simulink model "KiemnghiemDatathudc"  (R2021b)
settings: Solver=VariableStepAuto  StartTime=0.0  StopTime=10  RelTol=1e-3
InitFcn:
  | x_ref = 1; l_ref =0.2; l_ini = 0.6;
  | 
  | %ADRC' s parameter caculation
  | b0 = (ml+mc)/(mc*ml +mc*mt+ml*mt);k_ESO = 70;T_set  = 3;
  | 
  | s_cl = -5.85/T_set;
  | Kp   = s_cl^2;
  | Kd   = -2*s_cl;
  | 
  | s_ESO = k_ESO*s_cl;
  | l1        = -3*s_ESO;
  | l2        = 3*( s_ESO)^2;
  | l3        = -(s_ESO)^3;
  | 
  | %Observer
  | A = [-l1, 1, 0;
  |         -l2, 0, 1;
  |         -l3, 0, 0];
  | B = [0;
  |         b0;
  |         0];
  | L = [l1;
  |        l2;
  |        l3];
  | 
  | b1 = (mt+mc)/(mc*ml +mc*mt+ml*mt);k_ESO1 =100;T_set1  = 3;
  | s_cl1 = -5.85/T_set1;
  | Kp1   = s_cl1^2;
  | Kd1   = -2*s_cl1;
  | 
  | s_ESO1 = k_ESO1*s_cl1;
  | l11        = -3*s_ESO1;
  | l21        = 3*( s_ESO1)^2;
  | l31        = -(s_ESO1)^3;
  | 
  | %Observer
  | A1 = [-l11, 1, 0;
  |         -l21, 0, 1;
  |         -l31, 0, 0];
  | B1 = [0;
  |         b1;
  |         0];
  | L1 = [l11;
  |        l21;
  |        l31];
values from neighbouring files (symbols this model uses):
  g = 9.81    [Thong_so_double_pendulum.m]
undefined symbols (not defined in the file or in its folder): K_pso, mc, sigbuilder_block, T_pso, waof, waol
libraries: neural x95, simulink x11, simulink_extras x11
(part 1 of 6)
settings Model: Creator=Dao Hieu  LastModifiedBy=Admin

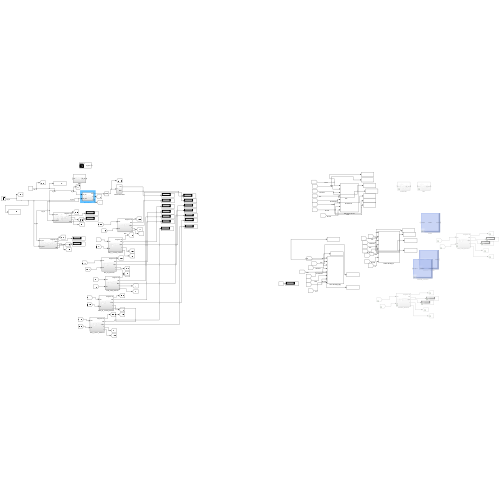
[thumbnail: Simulink's stored preview of the top-level diagram]
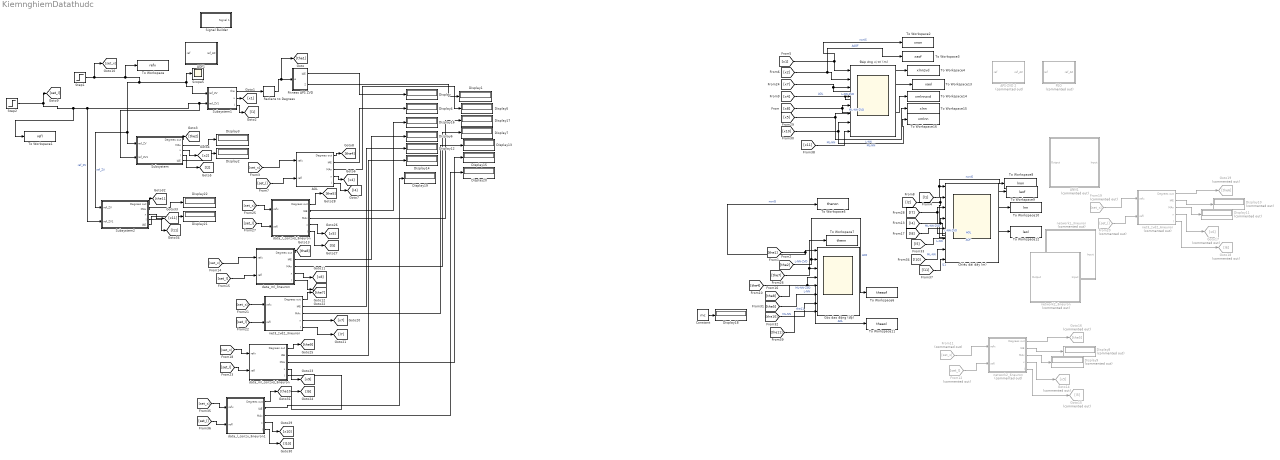
== system KiemnghiemDatathudc ==
  ANN1 : Subsystem  Commented=on
      mask help: Function Fitting Neural Network
      mask Display: e = 0.06;c1 = [120 150 230]/255;c2 = ([120 150 230]+0)/383;c3 = ([120 150 230]+128)/383;patch([0 1 1 0],[0 0 1 1],c1);patch([0 1 1 1-e 1-e 0+e],[0 0 1 1-e 0+e 0+e],c2);patch([0 0 1 1-e 0+e 0+e],[0 1 1 1-e 1-e 0+e],c3);plot([0 1 1 0 0],[0 0 1 1 0]);fprintf('NNET');port_label('input',1,' Input');port_label('output',1,'Output ');
  AOF1 : Subsystem
  AOL : Subsystem
  APS-ZVD 2 : Subsystem  Commented=on
  Chiều dài dây (m) : Scope  NumInputPorts=8
  Constant : Constant  Value=mc
  Display{,1..7,12..22} (19 alike) : Display
  Display{8..11} (4 alike) : Display  Commented=on
  Fitness APS ZVD : Subsystem
  From11 : From  Commented=on  GotoTag=set_x
  From12 : From  Commented=on  GotoTag=set_l
  From19 : From  Commented=on  GotoTag=set_x
  From20 : From  Commented=on  GotoTag=set_l
  Goto14 : Goto  Commented=on  GotoTag=x5
  Goto15 : Goto  Commented=on  GotoTag=l5
  Goto16 : Goto  Commented=on  GotoTag=the5
  Goto17 : Goto  Commented=on  GotoTag=x6
  Goto18 : Goto  Commented=on  GotoTag=l6
  Goto19 : Goto  Commented=on  GotoTag=the6
  Góc dao động (độ) : Scope  NumInputPorts=8
  PSO : Subsystem  Commented=on
  Radians to Degrees : simulink_extras/Transformations/Radians to Degrees
  Scope5 : Scope
  Signal Builder : Subsystem  Tag=STV Subsys  LoadFcn=sigbuilder_block('load');  StartFcn=sigbuilder_block('start');  StopFcn=sigbuilder_block('stop');  ClipboardFcn=sigbuilder_block('clipboard');  mask(Sigbuilder block){tuvar=[0:10]}
      mask help: Simulink:masks:SigbuilderBlock_MD
      mask init:
      | if ~strcmp(get_param(bdroot(gcbh),'SimulationStatus'),'stopped') tuvar = sigbuilder_block('maskInit'); end
      settings: CopyFcn=sigbuilder_block('copy');  DeleteFcn=sigbuilder_block('delete');  ModelCloseFcn=sigbuilder_block('modelClose');  PreSaveFcn=sigbuilder_block('preSave');  PauseFcn=sigbuilder_block('pause');  ContinueFcn=sigbuilder_block('continue');  NameChangeFcn=sigbuilder_block('namechange');  OpenFcn=sigbuilder_block('open',[420.6 144 550.8 400.2 ]);  CloseFcn=sigbuilder_block('close');
      mask Display: plot(0, 0, 100, 100,[2, 2, 32, 32, 2], [68, 8, 8, 68, 68],[32, 2], [38, 38], [32, 19, 2],[53, 60, 44], [32, 17, 17, 2],[16, 16, 31, 31]);txt = getActiveGroup(gcbh);text(2, 100, txt,'verticalAlignment', 'top');
  Step1 : Step  After=x_ref  SampleTime=0
  Step2 : Step  Before=l_ini  After=l_ref  SampleTime=0
  Subsystem : Subsystem
  Subsystem1 : Subsystem
  Subsystem2 : Subsystem
  To Workspace : ToWorkspace  VariableName=refx  SampleTime=0.001
  To Workspace1 : ToWorkspace  VariableName=refl  SampleTime=0.001
  To Workspace10 : ToWorkspace  VariableName=lnn  SampleTime=0.001
  To Workspace11 : ToWorkspace  VariableName=theaol  SampleTime=0.001
  To Workspace12 : ToWorkspace  VariableName=laol  SampleTime=0.001
  To Workspace13 : ToWorkspace  VariableName=xaol  SampleTime=0.001
  To Workspace14 : ToWorkspace  VariableName=xmlnnzvd  SampleTime=0.001
  To Workspace15 : ToWorkspace  VariableName=xlnn  SampleTime=0.001
  To Workspace16 : ToWorkspace  VariableName=xmlnn  SampleTime=0.001
  To Workspace2 : ToWorkspace  VariableName=xnon  SampleTime=0.001
  To Workspace3 : ToWorkspace  VariableName=xaof  SampleTime=0.001
  To Workspace4 : ToWorkspace  VariableName=xlnnzvd  SampleTime=0.001
  To Workspace5 : ToWorkspace  VariableName=thenon  SampleTime=0.001
  To Workspace6 : ToWorkspace  VariableName=theaof  SampleTime=0.001
  To Workspace7 : ToWorkspace  VariableName=thenn  SampleTime=0.001
  To Workspace8 : ToWorkspace  VariableName=lnon  SampleTime=0.001
  To Workspace9 : ToWorkspace  VariableName=laof  SampleTime=0.001
  data_l_conzv_3neuron1 : Subsystem
  data_l_conzvd_3neuron : Subsystem
  data_ml_3neuron : Subsystem
  data_ml_conzvd_3neuron : Subsystem
  net3_zvd2_3neuron : Subsystem
  net3_zvd2_6neuron : Subsystem  Commented=on
  network1_3neuron : Subsystem  Commented=on
      mask help: Custom Neural Network
      mask Display: e = 0.06;c1 = [120 150 230]/255;c2 = ([120 150 230]+0)/383;c3 = ([120 150 230]+128)/383;patch([0 1 1 0],[0 0 1 1],c1);patch([0 1 1 1-e 1-e 0+e],[0 0 1 1-e 0+e 0+e],c2);patch([0 0 1 1-e 0+e 0+e],[0 1 1 1-e 1-e 0+e],c3);plot([0 1 1 0 0],[0 0 1 1 0]);fprintf('NNET');port_label('input',1,' Input');port_label('output',1,'Output ');
  network2_3neuron : Subsystem  Commented=on
      mask help: Custom Neural Network
      mask Display: e = 0.06;c1 = [120 150 230]/255;c2 = ([120 150 230]+0)/383;c3 = ([120 150 230]+128)/383;patch([0 1 1 0],[0 0 1 1],c1);patch([0 1 1 1-e 1-e 0+e],[0 0 1 1-e 0+e 0+e],c2);patch([0 0 1 1-e 0+e 0+e],[0 1 1 1-e 1-e 0+e],c3);plot([0 1 1 0 0],[0 0 1 1 0]);fprintf('NNET');port_label('input',1,' Input');port_label('output',1,'Output ');
  network2_6neuron : Subsystem  Commented=on
  Đáp ứng vị trí (m) : Scope  NumInputPorts=8
  wires:
  Radians to Degrees/1 -> [the1], Fitness APS ZVD/1(e)
  Fitness APS ZVD/2(MAx) -> Display1/1
  Fitness APS ZVD/1(IAE) -> Display/1
  Subsystem1/1(the) -> Radians to Degrees/1
  [x2] -> Đáp ứng vị trí (m)/2, To Workspace3/1  "AAOF"
  [x1] -> To Workspace2/1, Đáp ứng vị trí (m)/1  "nonIS"
  [the2] -> To Workspace6/1, Góc dao động (độ)/2  "AOF"
  [the1] -> To Workspace5/1, Góc dao động (độ)/1  "nonIS"
  [l2] -> To Workspace9/1, Chiều dài dây (m)/2  "AOF"
  [l1] -> To Workspace8/1, Chiều dài dây (m)/1  "nonIS"
  Subsystem1/2(x) -> [x1]
  Subsystem1/3(l) -> [l1]
  From11/1 -> network2_6neuron/1(refx)
  network2_6neuron/1(Degrees out) -> Goto16/1
  network2_6neuron/2(IAE) -> Display8/1
  network2_6neuron/3(MAx) -> Display9/1
  network2_6neuron/4(x) -> Goto14/1
  network2_6neuron/5(l) -> Goto15/1
  From12/1 -> network2_6neuron/2(refl)
  net3_zvd2_6neuron/5(l) -> Goto18/1
  net3_zvd2_6neuron/1(Degrees out) -> Goto19/1
  net3_zvd2_6neuron/4(x) -> Goto17/1
  net3_zvd2_6neuron/3(MAx) -> Display11/1
  net3_zvd2_6neuron/2(IAE) -> Display10/1
  From19/1 -> net3_zvd2_6neuron/1(refx)
  From20/1 -> net3_zvd2_6neuron/2(refl)
  net3_zvd2_3neuron/5(l) -> [l7]
  net3_zvd2_3neuron/1(Degrees out) -> [the7]
  net3_zvd2_3neuron/4(x) -> [x7]
  net3_zvd2_3neuron/3(MAx) -> Display13/1
  net3_zvd2_3neuron/2(IAE) -> Display12/1
  [set_x] -> net3_zvd2_3neuron/1(refx)
  [set_l] -> net3_zvd2_3neuron/2(refl)
  [x7] -> To Workspace4/1, Đáp ứng vị trí (m)/3  "L-NN-ZVD"
  [l7] -> To Workspace10/1, Chiều dài dây (m)/3  "L-NN-ZVD"
  [the7] -> To Workspace7/1, Góc dao động (độ)/3  "L-NN-ZVD"
  AOL/2(IAE) -> Display4/1
  AOL/4(x) -> [x4]
  AOL/5(l) -> [l4]
  AOL/3(MAx) -> Display5/1
  [set_l] -> AOL/2(refl)
  AOL/1(Degrees out) -> [the4]
  [set_x] -> AOL/1(refx)
  [x4] -> To Workspace13/1, Đáp ứng vị trí (m)/4  "AOL"
  [the4] -> To Workspace11/1, Góc dao động (độ)/4  "AOL"
  [l4] -> To Workspace12/1, Chiều dài dây (m)/4  "AOL"
  [set_l] -> data_ml_3neuron/2(refl)
  [set_x] -> data_ml_3neuron/1(refx)
  data_ml_3neuron/1(Degrees out) -> [the8]
  data_ml_3neuron/3(MAx) -> Display7/1
  data_ml_3neuron/5(l) -> [l8]
  data_ml_3neuron/2(IAE) -> Display6/1
  data_ml_3neuron/4(x) -> [x8]
  [x8] -> To Workspace14/1, Đáp ứng vị trí (m)/5  "ML-NN-ZVD"
  [the8] -> Góc dao động (độ)/5  "ML-NN-ZVD"
  [l8] -> Chiều dài dây (m)/5  "ML-NN-ZVD"
  [set_l] -> data_ml_conzvd_3neuron/2(refl)
  [set_x] -> data_ml_conzvd_3neuron/1(refx)
  data_ml_conzvd_3neuron/1(Degrees out) -> [the9]
  data_ml_conzvd_3neuron/3(MAx) -> Display15/1
  data_ml_conzvd_3neuron/5(l) -> [l9]
  data_ml_conzvd_3neuron/2(IAE) -> Display14/1
  data_ml_conzvd_3neuron/4(x) -> [x9]
  [set_l] -> data_l_conzvd_3neuron/2(refl)
  [set_x] -> data_l_conzvd_3neuron/1(refx)
  data_l_conzvd_3neuron/1(Degrees out) -> [the5]
  data_l_conzvd_3neuron/3(MAx) -> Display17/1
  data_l_conzvd_3neuron/5(l) -> [l5]
  data_l_conzvd_3neuron/2(IAE) -> Display16/1
  data_l_conzvd_3neuron/4(x) -> [x5]
  [l5] -> Chiều dài dây (m)/6  "L-NN"
  [l10] -> Chiều dài dây (m)/7  "ML-NN"
  [the5] -> Góc dao động (độ)/6  "L-NN"
  [the10] -> Góc dao động (độ)/7  "ML-NN"
  [x5] -> To Workspace15/1, Đáp ứng vị trí (m)/6  "L-NN"
  [x10] -> To Workspace16/1, Đáp ứng vị trí (m)/7  "ML-NN"
  Constant/1 -> Display18/1
  data_l_conzv_3neuron1/5(l) -> [l10]
  data_l_conzv_3neuron1/2(IAE) -> Display19/1
  data_l_conzv_3neuron1/4(x) -> [x10]
  [set_x] -> data_l_conzv_3neuron1/1(refx)
  [set_l] -> data_l_conzv_3neuron1/2(refl)
  data_l_conzv_3neuron1/1(Degrees out) -> [the10]
  data_l_conzv_3neuron1/3(MAx) -> Display20/1
  Subsystem/1(Degrees out) -> [the2]
  Subsystem/2(MAx) -> Display3/1
  Subsystem/3(x) -> [x2]
  Subsystem/4(l) -> [l2]
  Subsystem/5(IAE) -> Display2/1
  Subsystem2/4(l) -> [l11]
  Subsystem2/1(Degrees out) -> [the11]
  Step1/1 -> To Workspace/1, Subsystem2/1(ref_ZV), Subsystem/1(ref_ZV), Subsystem1/1(ref_ZV), Scope5/1, [set_x]  "ref_ZV"
  Step2/1 -> Subsystem/2(ref_ZV1), Subsystem1/2(ref_ZV1), Subsystem2/2(ref_ZV1), To Workspace1/1, [set_l]  "ref_ZV"
  Subsystem2/2(MAx) -> Display22/1
  Subsystem2/3(x) -> [x11]
  Subsystem2/5(IAE) -> Display21/1
  [l11] -> Chiều dài dây (m)/8  "l11"
  [x11] -> Đáp ứng vị trí (m)/8  "ML-NN"
  [the11] -> Góc dao động (độ)/8  "the11"

== system KiemnghiemDatathudc/ANN1 ==
  Input : Inport  PortDimensions=1
      mask Display: e = 0.06;c1 = [120 230 180]/255;c2 = ([120 230 180]+0)/(256+128);c3 = ([120 230 180]+128)/(256+128);patch([0 1 1 0],[0 0 1 1],c1);patch([0 1 1 1-e 1-e 0+e],[0 0 1 1-e 0+e 0+e],c2);patch([0 0 1 1-e 0+e 0+e],[0 1 1 1-e 1-e 0+e],c3);plot([0 1 1 0 0],[0 0 1 1 0]);
  Layer 1 : Subsystem
      mask Display: e = 0.06;c1 = [120 150 230]/255;c2 = ([120 150 230]+0)/383;c3 = ([120 150 230]+128)/383;patch([0 1 1 0],[0 0 1 1],c1);patch([0 1 1 1-e 1-e 0+e],[0 0 1 1-e 0+e 0+e],c2);patch([0 0 1 1-e 0+e 0+e],[0 1 1 1-e 1-e 0+e],c3);plot([0 1 1 0 0],[0 0 1 1 0]);
  Layer 2 : Subsystem
      mask Display: e = 0.06;c1 = [120 150 230]/255;c2 = ([120 150 230]+0)/383;c3 = ([120 150 230]+128)/383;patch([0 1 1 0],[0 0 1 1],c1);patch([0 1 1 1-e 1-e 0+e],[0 0 1 1-e 0+e 0+e],c2);patch([0 0 1 1-e 0+e 0+e],[0 1 1 1-e 1-e 0+e],c3);plot([0 1 1 0 0],[0 0 1 1 0]);
  Process Input 1 : Subsystem
      mask Display: e = 0.06;c1 = [120 150 230]/255;c2 = ([120 150 230]+0)/383;c3 = ([120 150 230]+128)/383;patch([0 1 1 0],[0 0 1 1],c1);patch([0 1 1 1-e 1-e 0+e],[0 0 1 1-e 0+e 0+e],c2);patch([0 0 1 1-e 0+e 0+e],[0 1 1 1-e 1-e 0+e],c3);plot([0 1 1 0 0],[0 0 1 1 0]);
  Process Output 1 : Subsystem
      mask Display: e = 0.06;c1 = [120 150 230]/255;c2 = ([120 150 230]+0)/383;c3 = ([120 150 230]+128)/383;patch([0 1 1 0],[0 0 1 1],c1);patch([0 1 1 1-e 1-e 0+e],[0 0 1 1-e 0+e 0+e],c2);patch([0 0 1 1-e 0+e 0+e],[0 1 1 1-e 1-e 0+e],c3);plot([0 1 1 0 0],[0 0 1 1 0]);
  Output : Outport  InitialOutput=[0;0]
      mask Display: e = 0.06;c1 = [120 230 180]/255;c2 = ([120 230 180]+0)/(256+128);c3 = ([120 230 180]+128)/(256+128);patch([0 1 1 0],[0 0 1 1],c1);patch([0 1 1 1-e 1-e 0+e],[0 0 1 1-e 0+e 0+e],c2);patch([0 0 1 1-e 0+e 0+e],[0 1 1 1-e 1-e 0+e],c3);plot([0 1 1 0 0],[0 0 1 1 0]);
  wires:
  Input/1 -> Process Input 1/1(x)
  Process Output 1/1(y) -> Output/1
  Process Input 1/1(p) -> Layer 1/1("p{1}")
  Layer 1/1("a{1}") -> [feedback1]
  [feedback1] -> Layer 2/1("a{1} ")
  Layer 2/1("a{2}") -> Process Output 1/1(a)

== system KiemnghiemDatathudc/AOF1 ==
  ref : Inport
  Gain : Gain  Gain=0.5
  Gain1 : Gain  Gain=0.5
  Sum : Sum
  Transport Delay : TransportDelay  DelayTime=pi/sqrt(g/0.4)
  ref_AZ : Outport
  wires:
  Gain1/1 -> Transport Delay/1
  Gain/1 -> Sum/1
  Transport Delay/1 -> Sum/2
  Sum/1 -> ref_AZ/1
  ref/1 -> Gain/1, Gain1/1

== system KiemnghiemDatathudc/AOL ==
  refx : Inport
  refl : Inport  Port=2
  AOL : Subsystem
  Fitness APS ZVD4 : Subsystem
  Radians to Degrees4 : simulink_extras/Transformations/Radians to Degrees
  Subsystem5 : Subsystem
  Degrees out : Outport
  IAE : Outport  Port=2
  MAx : Outport  Port=3
  x : Outport  Port=4
  l : Outport  Port=5
  wires:
  refl/1 -> Subsystem5/2(ref_ZV1)
  Subsystem5/1(the) -> Radians to Degrees4/1
  Fitness APS ZVD4/1(IAE) -> IAE/1
  Radians to Degrees4/1 -> Degrees out/1, Fitness APS ZVD4/1(e)
  Subsystem5/3(l) -> l/1
  AOL/1(ref_AZ) -> Subsystem5/1(ref_ZV)  "ref_ZV"
  refx/1 -> AOL/1(ref)
  Subsystem5/2(x) -> x/1
  Fitness APS ZVD4/2(MAx) -> MAx/1

== system KiemnghiemDatathudc/APS-ZVD 2 ==
  ref : Inport
  Gain : Gain
  Gain1 : Gain  Gain=-1
  Gain2 : Gain
  Sum : Sum  Inputs=+++
  Transport Delay : TransportDelay  DelayTime=0.213149037770351
  Transport Delay1 : TransportDelay  DelayTime=0.426777072460345
  ref_AZ : Outport
  wires:
  Gain1/1 -> Transport Delay/1
  Gain/1 -> Sum/1
  Transport Delay/1 -> Sum/2
  Sum/1 -> ref_AZ/1
  ref/1 -> Gain/1, Gain2/1, Gain1/1
  Gain2/1 -> Transport Delay1/1
  Transport Delay1/1 -> Sum/3

== system KiemnghiemDatathudc/Fitness APS ZVD ==
  e : Inport
  Abs : Abs
  Abs1 : Abs
  Integrator : Integrator
  MinMax Running Resettable : simulink/Math Operations/MinMax Running Resettable  Function=max  vinit=0.0
  Step : Step  Time=0.000001  Before=1  After=0  SampleTime=0
  IAE : Outport
  MAx : Outport  Port=2
  wires:
  Abs/1 -> Integrator/1
  Abs1/1 -> MinMax Running Resettable/1
  Step/1 -> MinMax Running Resettable/2
  e/1 -> Abs/1, Abs1/1
  Integrator/1 -> IAE/1
  MinMax Running Resettable/1 -> MAx/1

== system KiemnghiemDatathudc/PSO ==
  ref : Inport
  Gain : Gain  Gain=1/(K_pso^2+2*K_pso+1)
  Gain1 : Gain  Gain=2*K_pso/(K_pso^2+2*K_pso+1)
  Gain2 : Gain  Gain=K_pso^2/(K_pso^2+2*K_pso+1)
  Sum : Sum  Inputs=+++
  Transport Delay : TransportDelay  DelayTime=T_pso
  Transport Delay1 : TransportDelay  DelayTime=2*T_pso
  ref_AZ : Outport
  wires:
  Gain1/1 -> Transport Delay/1
  Gain/1 -> Sum/1
  Transport Delay/1 -> Sum/2
  Sum/1 -> ref_AZ/1
  ref/1 -> Gain/1, Gain2/1, Gain1/1
  Gain2/1 -> Transport Delay1/1
  Transport Delay1/1 -> Sum/3

== system KiemnghiemDatathudc/Signal Builder ==
  Demux : Demux  Tag=STV Demux  Outputs=1
      settings: DisplayOption=none
  FromWs : FromWorkspace  Tag=STV FromWs  VariableName=tuvar
      SigBuilderData=|
      | common.afterFinalStr = 'Extrapolate'
      | common.sampleTime = 0
      | dataSet.timeRange = [0 10]
      | dataSet.name = 'Group 1'
      | sbobj.Groups.Name = 'Group 1'
      | sbobj.Groups.Signals.Name = 'Signal 1'
      | sbobj.Groups.Signals.XData = [0 1 1 3 3 10]
      | sbobj.Groups.Signals.YData = [0.6 0.6 0.2 0.2 0.6 0.6]
  Signal 1 : Outport  Tag=STV Outport
  wires:
  Demux/1 -> Signal 1/1
  FromWs/1 -> Demux/1

== system KiemnghiemDatathudc/Subsystem ==
  ref_ZV : Inport
  ref_ZV1 : Inport  Port=2
  AOF : Subsystem
  AOF2 : Subsystem
  Constant : Constant  Value=l_ini
  Constant1 : Constant  Value=l_ini
  Fitness APS ZVD1 : Subsystem
  Radians to Degrees1 : simulink_extras/Transformations/Radians to Degrees
  Scope : Scope  NumInputPorts=2
  Subsystem5 : Subsystem
  Subtract : Sum  Inputs=+-
  Sum : Sum  Inputs=|++
  Degrees out : Outport
  MAx : Outport  Port=2
  x : Outport  Port=3
  l : Outport  Port=4
  IAE : Outport  Port=5
  wires:
  Radians to Degrees1/1 -> Degrees out/1, Fitness APS ZVD1/1(e)
  Subsystem5/2(x) -> x/1
  ref_ZV1/1 -> Subtract/1, Scope/1
  Subsystem5/3(l) -> l/1
  Subsystem5/1(the) -> Radians to Degrees1/1
  AOF2/1(ref_AZ) -> Sum/1  "ref_ZV"
  AOF/1(ref_AZ) -> Subsystem5/1(ref_ZV)  "ref_ZV"
  Fitness APS ZVD1/1(IAE) -> IAE/1
  Fitness APS ZVD1/2(MAx) -> MAx/1
  ref_ZV/1 -> AOF/1(ref)
  Subtract/1 -> AOF2/1(ref)
  Constant/1 -> Subtract/2
  Sum/1 -> Subsystem5/2(ref_ZV1), Scope/2
  Constant1/1 -> Sum/2

== system KiemnghiemDatathudc/Subsystem1 ==
  ref_ZV : Inport
  ref_ZV1 : Inport  Port=2
  "ADRC " : Subsystem
  ADRC 1 : Subsystem
  Constant : Constant  Value=mc
  Gain : Gain  Gain=1/3
  Subsystem : Subsystem
  the : Outport
  x : Outport  Port=2
  l : Outport  Port=3
  wires:
  Subsystem/1(x) -> x/1, "ADRC "/2(x)  "Position"
  ADRC 1/1(u) -> Subsystem/2(ul)  "ADRC"
  Subsystem/3(the) -> Gain/1
  Subsystem/2(l) -> ADRC 1/2(x), l/1  "Length"
  "ADRC "/1(u) -> Subsystem/1(ut)  "ADRC"
  ref_ZV1/1 -> ADRC 1/1(ref)
  ref_ZV/1 -> "ADRC "/1(ref)
  Gain/1 -> the/1
  Constant/1 -> Subsystem/3(mc)

== system KiemnghiemDatathudc/Subsystem2 ==
  ref_ZV : Inport
  ref_ZV1 : Inport  Port=2
  AOF : Subsystem
  Fitness APS ZVD1 : Subsystem
  Radians to Degrees1 : simulink_extras/Transformations/Radians to Degrees
  Subsystem5 : Subsystem
  Degrees out : Outport
  MAx : Outport  Port=2
  x : Outport  Port=3
  l : Outport  Port=4
  IAE : Outport  Port=5
  wires:
  Radians to Degrees1/1 -> Degrees out/1, Fitness APS ZVD1/1(e)
  Subsystem5/2(x) -> x/1
  Subsystem5/3(l) -> l/1
  Subsystem5/1(the) -> Radians to Degrees1/1
  ref_ZV1/1 -> Subsystem5/2(ref_ZV1)  "ref_ZV"
  AOF/1(ref_AZ) -> Subsystem5/1(ref_ZV)  "ref_ZV"
  Fitness APS ZVD1/1(IAE) -> IAE/1
  Fitness APS ZVD1/2(MAx) -> MAx/1
  ref_ZV/1 -> AOF/1(ref)

== system KiemnghiemDatathudc/data_l_conzv_3neuron1 ==
  refx : Inport
  refl : Inport  Port=2
  Custom Neural Network1 : Subsystem
      mask help: Custom Neural Network
      mask Display: e = 0.06;c1 = [120 150 230]/255;c2 = ([120 150 230]+0)/383;c3 = ([120 150 230]+128)/383;patch([0 1 1 0],[0 0 1 1],c1);patch([0 1 1 1-e 1-e 0+e],[0 0 1 1-e 0+e 0+e],c2);patch([0 0 1 1-e 0+e 0+e],[0 1 1 1-e 1-e 0+e],c3);plot([0 1 1 0 0],[0 0 1 1 0]);fprintf('NNET');port_label('input',1,' Input');port_label('output',1,'Output ');
  Fitness APS ZVD4 : Subsystem
  Radians to Degrees4 : simulink_extras/Transformations/Radians to Degrees
  Scope : Scope
  Subsystem5 : Subsystem
  ZV3 : Subsystem
  Degrees out : Outport
  IAE : Outport  Port=2
  MAx : Outport  Port=3
  x : Outport  Port=4
  l : Outport  Port=5
  wires:
  refl/1 -> Subsystem5/2(ref_ZV1)
  Subsystem5/1(the) -> Radians to Degrees4/1
  Fitness APS ZVD4/1(IAE) -> IAE/1
  Radians to Degrees4/1 -> Degrees out/1, Fitness APS ZVD4/1(e)
  Subsystem5/3(l) -> Custom Neural Network1/1(Input), l/1
  ZV3/1(ref_AZ) -> Scope/1, Subsystem5/1(ref_ZV)  "ref_ZV"
  refx/1 -> ZV3/1(ref)
  Subsystem5/2(x) -> x/1
  Fitness APS ZVD4/2(MAx) -> MAx/1
  Custom Neural Network1/1(Output) -> ZV3/2(Input)

== system KiemnghiemDatathudc/data_l_conzvd_3neuron ==
  refx : Inport
  refl : Inport  Port=2
  Custom Neural Network : Subsystem
      mask help: Custom Neural Network
      mask Display: e = 0.06;c1 = [120 150 230]/255;c2 = ([120 150 230]+0)/383;c3 = ([120 150 230]+128)/383;patch([0 1 1 0],[0 0 1 1],c1);patch([0 1 1 1-e 1-e 0+e],[0 0 1 1-e 0+e 0+e],c2);patch([0 0 1 1-e 0+e 0+e],[0 1 1 1-e 1-e 0+e],c3);plot([0 1 1 0 0],[0 0 1 1 0]);fprintf('NNET');port_label('input',1,' Input');port_label('output',1,'Output ');
  Demux2 : Demux  Outputs=2
  Fitness APS ZVD4 : Subsystem
  Radians to Degrees4 : simulink_extras/Transformations/Radians to Degrees
  Subsystem5 : Subsystem
  ZVD3 : Subsystem
  Degrees out : Outport
  IAE : Outport  Port=2
  MAx : Outport  Port=3
  x : Outport  Port=4
  l : Outport  Port=5
  wires:
  refl/1 -> Subsystem5/2(ref_ZV1)
  Subsystem5/1(the) -> Radians to Degrees4/1
  Fitness APS ZVD4/1(IAE) -> IAE/1
  Radians to Degrees4/1 -> Degrees out/1, Fitness APS ZVD4/1(e)
  Subsystem5/3(l) -> ZVD3/4(Input1), Custom Neural Network/1(Input), l/1
  Demux2/1 -> ZVD3/2(Input)
  ZVD3/1(ref_AZ) -> Subsystem5/1(ref_ZV)  "ref_ZV"
  Demux2/2 -> ZVD3/3(Input2)
  Custom Neural Network/1(Output) -> Demux2/1
  refx/1 -> ZVD3/1(ref)
  Subsystem5/2(x) -> x/1
  Fitness APS ZVD4/2(MAx) -> MAx/1

== system KiemnghiemDatathudc/data_ml_3neuron ==
  refx : Inport
  refl : Inport  Port=2
  Constant : Constant  Value=mc
  Custom Neural Network : Subsystem
      mask help: Custom Neural Network
      mask Display: e = 0.06;c1 = [120 150 230]/255;c2 = ([120 150 230]+0)/383;c3 = ([120 150 230]+128)/383;patch([0 1 1 0],[0 0 1 1],c1);patch([0 1 1 1-e 1-e 0+e],[0 0 1 1-e 0+e 0+e],c2);patch([0 0 1 1-e 0+e 0+e],[0 1 1 1-e 1-e 0+e],c3);plot([0 1 1 0 0],[0 0 1 1 0]);fprintf('NNET');port_label('input',1,' Input');port_label('output',1,'Output ');
  Demux2 : Demux  Outputs=2
  Fitness APS ZVD4 : Subsystem
  Mux : Mux  Inputs=2
  Radians to Degrees4 : simulink_extras/Transformations/Radians to Degrees
  Subsystem5 : Subsystem
  ZVD3 : Subsystem
  Degrees out : Outport
  IAE : Outport  Port=2
  MAx : Outport  Port=3
  x : Outport  Port=4
  l : Outport  Port=5
  wires:
  refl/1 -> Subsystem5/2(ref_ZV1)
  Subsystem5/1(the) -> Radians to Degrees4/1
  Fitness APS ZVD4/1(IAE) -> IAE/1
  Radians to Degrees4/1 -> Degrees out/1, Fitness APS ZVD4/1(e)
  Subsystem5/3(l) -> Mux/2, l/1
  Demux2/1 -> ZVD3/2(K)
  ZVD3/1(ref_AZ) -> Subsystem5/1(ref_ZV)  "ref_ZV"
  Demux2/2 -> ZVD3/3(T)
  Custom Neural Network/1(Output) -> Demux2/1
  refx/1 -> ZVD3/1(ref)
  Subsystem5/2(x) -> x/1
  Fitness APS ZVD4/2(MAx) -> MAx/1
  Mux/1 -> Custom Neural Network/1(Input)
  Constant/1 -> Mux/1

== system KiemnghiemDatathudc/data_ml_conzvd_3neuron ==
  refx : Inport
  refl : Inport  Port=2
  Constant : Constant  Value=mc
  Custom Neural Network : Subsystem
      mask help: Custom Neural Network
      mask Display: e = 0.06;c1 = [120 150 230]/255;c2 = ([120 150 230]+0)/383;c3 = ([120 150 230]+128)/383;patch([0 1 1 0],[0 0 1 1],c1);patch([0 1 1 1-e 1-e 0+e],[0 0 1 1-e 0+e 0+e],c2);patch([0 0 1 1-e 0+e 0+e],[0 1 1 1-e 1-e 0+e],c3);plot([0 1 1 0 0],[0 0 1 1 0]);fprintf('NNET');port_label('input',1,' Input');port_label('output',1,'Output ');
  Demux2 : Demux  Outputs=2
  Fitness APS ZVD4 : Subsystem
  Mux : Mux  Inputs=2
  Radians to Degrees4 : simulink_extras/Transformations/Radians to Degrees
  Subsystem5 : Subsystem
  ZVD3 : Subsystem
  Degrees out : Outport
  IAE : Outport  Port=2
  MAx : Outport  Port=3
  x : Outport  Port=4
  l : Outport  Port=5
  wires:
  refl/1 -> Subsystem5/2(ref_ZV1)
  Subsystem5/1(the) -> Radians to Degrees4/1
  Fitness APS ZVD4/1(IAE) -> IAE/1
  Radians to Degrees4/1 -> Degrees out/1, Fitness APS ZVD4/1(e)
  Subsystem5/3(l) -> Mux/2, l/1
  Demux2/1 -> ZVD3/2(Input)
  ZVD3/1(ref_AZ) -> Subsystem5/1(ref_ZV)  "ref_ZV"
  Demux2/2 -> ZVD3/3(Input1)
  Custom Neural Network/1(Output) -> Demux2/1
  refx/1 -> ZVD3/1(ref)
  Subsystem5/2(x) -> x/1
  Fitness APS ZVD4/2(MAx) -> MAx/1
  Mux/1 -> Custom Neural Network/1(Input)
  Constant/1 -> Mux/1

== system KiemnghiemDatathudc/net3_zvd2_3neuron ==
  refx : Inport
  refl : Inport  Port=2
  Demux2 : Demux  Outputs=2
  Fitness APS ZVD4 : Subsystem
  Radians to Degrees4 : simulink_extras/Transformations/Radians to Degrees
  Scope : Scope
  Subsystem5 : Subsystem
  ZVD3 : Subsystem
  net3_zvd2_3neuron : Subsystem
      mask help: Custom Neural Network
      mask Display: e = 0.06;c1 = [120 150 230]/255;c2 = ([120 150 230]+0)/383;c3 = ([120 150 230]+128)/383;patch([0 1 1 0],[0 0 1 1],c1);patch([0 1 1 1-e 1-e 0+e],[0 0 1 1-e 0+e 0+e],c2);patch([0 0 1 1-e 0+e 0+e],[0 1 1 1-e 1-e 0+e],c3);plot([0 1 1 0 0],[0 0 1 1 0]);fprintf('NNET');port_label('input',1,' Input');port_label('output',1,'Output ');
  Degrees out : Outport
  IAE : Outport  Port=2
  MAx : Outport  Port=3
  x : Outport  Port=4
  l : Outport  Port=5
  wires:
  refl/1 -> Subsystem5/2(ref_ZV1)
  Subsystem5/1(the) -> Radians to Degrees4/1
  Fitness APS ZVD4/1(IAE) -> IAE/1
  Radians to Degrees4/1 -> Degrees out/1, Fitness APS ZVD4/1(e)
  Subsystem5/3(l) -> net3_zvd2_3neuron/1(Input), l/1
  Demux2/1 -> ZVD3/2(K)
  ZVD3/1(ref_AZ) -> Scope/1, Subsystem5/1(ref_ZV)  "ref_ZV"
  Demux2/2 -> ZVD3/3(T)
  net3_zvd2_3neuron/1(Output) -> Demux2/1
  refx/1 -> ZVD3/1(ref)
  Subsystem5/2(x) -> x/1
  Fitness APS ZVD4/2(MAx) -> MAx/1

== system KiemnghiemDatathudc/net3_zvd2_6neuron ==
  refx : Inport
  refl : Inport  Port=2
  Demux2 : Demux  Outputs=2
  Fitness APS ZVD4 : Subsystem
  Radians to Degrees4 : simulink_extras/Transformations/Radians to Degrees
  Subsystem5 : Subsystem
  ZVD3 : Subsystem
  net3_zvd2_6neuron : Subsystem
      mask help: Custom Neural Network
      mask Display: e = 0.06;c1 = [120 150 230]/255;c2 = ([120 150 230]+0)/383;c3 = ([120 150 230]+128)/383;patch([0 1 1 0],[0 0 1 1],c1);patch([0 1 1 1-e 1-e 0+e],[0 0 1 1-e 0+e 0+e],c2);patch([0 0 1 1-e 0+e 0+e],[0 1 1 1-e 1-e 0+e],c3);plot([0 1 1 0 0],[0 0 1 1 0]);fprintf('NNET');port_label('input',1,' Input');port_label('output',1,'Output ');
  Degrees out : Outport
  IAE : Outport  Port=2
  MAx : Outport  Port=3
  x : Outport  Port=4
  l : Outport  Port=5
  wires:
  refl/1 -> Subsystem5/2(ref_ZV1)
  Subsystem5/1(the) -> Radians to Degrees4/1
  Fitness APS ZVD4/1(IAE) -> IAE/1
  Radians to Degrees4/1 -> Degrees out/1, Fitness APS ZVD4/1(e)
  Subsystem5/3(l) -> net3_zvd2_6neuron/1(Input), l/1
  Demux2/1 -> ZVD3/2(K)
  ZVD3/1(ref_AZ) -> Subsystem5/1(ref_ZV)  "ref_ZV"
  Demux2/2 -> ZVD3/3(T)
  net3_zvd2_6neuron/1(Output) -> Demux2/1
  refx/1 -> ZVD3/1(ref)
  Subsystem5/2(x) -> x/1
  Fitness APS ZVD4/2(MAx) -> MAx/1

== system KiemnghiemDatathudc/network1_3neuron ==
  Input : Inport  PortDimensions=1
      mask Display: e = 0.06;c1 = [120 230 180]/255;c2 = ([120 230 180]+0)/(256+128);c3 = ([120 230 180]+128)/(256+128);patch([0 1 1 0],[0 0 1 1],c1);patch([0 1 1 1-e 1-e 0+e],[0 0 1 1-e 0+e 0+e],c2);patch([0 0 1 1-e 0+e 0+e],[0 1 1 1-e 1-e 0+e],c3);plot([0 1 1 0 0],[0 0 1 1 0]);
  Layer 1 : Subsystem
      mask Display: e = 0.06;c1 = [120 150 230]/255;c2 = ([120 150 230]+0)/383;c3 = ([120 150 230]+128)/383;patch([0 1 1 0],[0 0 1 1],c1);patch([0 1 1 1-e 1-e 0+e],[0 0 1 1-e 0+e 0+e],c2);patch([0 0 1 1-e 0+e 0+e],[0 1 1 1-e 1-e 0+e],c3);plot([0 1 1 0 0],[0 0 1 1 0]);
  Layer 2 : Subsystem
      mask Display: e = 0.06;c1 = [120 150 230]/255;c2 = ([120 150 230]+0)/383;c3 = ([120 150 230]+128)/383;patch([0 1 1 0],[0 0 1 1],c1);patch([0 1 1 1-e 1-e 0+e],[0 0 1 1-e 0+e 0+e],c2);patch([0 0 1 1-e 0+e 0+e],[0 1 1 1-e 1-e 0+e],c3);plot([0 1 1 0 0],[0 0 1 1 0]);
  Process Input 1 : Subsystem
      mask Display: e = 0.06;c1 = [120 150 230]/255;c2 = ([120 150 230]+0)/383;c3 = ([120 150 230]+128)/383;patch([0 1 1 0],[0 0 1 1],c1);patch([0 1 1 1-e 1-e 0+e],[0 0 1 1-e 0+e 0+e],c2);patch([0 0 1 1-e 0+e 0+e],[0 1 1 1-e 1-e 0+e],c3);plot([0 1 1 0 0],[0 0 1 1 0]);
  Process Output 1 : Subsystem
      mask Display: e = 0.06;c1 = [120 150 230]/255;c2 = ([120 150 230]+0)/383;c3 = ([120 150 230]+128)/383;patch([0 1 1 0],[0 0 1 1],c1);patch([0 1 1 1-e 1-e 0+e],[0 0 1 1-e 0+e 0+e],c2);patch([0 0 1 1-e 0+e 0+e],[0 1 1 1-e 1-e 0+e],c3);plot([0 1 1 0 0],[0 0 1 1 0]);
  Output : Outport  InitialOutput=[0;0]
      mask Display: e = 0.06;c1 = [120 230 180]/255;c2 = ([120 230 180]+0)/(256+128);c3 = ([120 230 180]+128)/(256+128);patch([0 1 1 0],[0 0 1 1],c1);patch([0 1 1 1-e 1-e 0+e],[0 0 1 1-e 0+e 0+e],c2);patch([0 0 1 1-e 0+e 0+e],[0 1 1 1-e 1-e 0+e],c3);plot([0 1 1 0 0],[0 0 1 1 0]);
  wires:
  Input/1 -> Process Input 1/1(x)
  Process Output 1/1(y) -> Output/1
  Process Input 1/1(p) -> Layer 1/1("p{1}")
  Layer 1/1("a{1}") -> [feedback1]
  [feedback1] -> Layer 2/1("a{1} ")
  Layer 2/1("a{2}") -> Process Output 1/1(a)

== system KiemnghiemDatathudc/network2_3neuron ==
  Input : Inport  PortDimensions=1
      mask Display: e = 0.06;c1 = [120 230 180]/255;c2 = ([120 230 180]+0)/(256+128);c3 = ([120 230 180]+128)/(256+128);patch([0 1 1 0],[0 0 1 1],c1);patch([0 1 1 1-e 1-e 0+e],[0 0 1 1-e 0+e 0+e],c2);patch([0 0 1 1-e 0+e 0+e],[0 1 1 1-e 1-e 0+e],c3);plot([0 1 1 0 0],[0 0 1 1 0]);
  Layer 1 : Subsystem
      mask Display: e = 0.06;c1 = [120 150 230]/255;c2 = ([120 150 230]+0)/383;c3 = ([120 150 230]+128)/383;patch([0 1 1 0],[0 0 1 1],c1);patch([0 1 1 1-e 1-e 0+e],[0 0 1 1-e 0+e 0+e],c2);patch([0 0 1 1-e 0+e 0+e],[0 1 1 1-e 1-e 0+e],c3);plot([0 1 1 0 0],[0 0 1 1 0]);
  Layer 2 : Subsystem
      mask Display: e = 0.06;c1 = [120 150 230]/255;c2 = ([120 150 230]+0)/383;c3 = ([120 150 230]+128)/383;patch([0 1 1 0],[0 0 1 1],c1);patch([0 1 1 1-e 1-e 0+e],[0 0 1 1-e 0+e 0+e],c2);patch([0 0 1 1-e 0+e 0+e],[0 1 1 1-e 1-e 0+e],c3);plot([0 1 1 0 0],[0 0 1 1 0]);
  Process Input 1 : Subsystem
      mask Display: e = 0.06;c1 = [120 150 230]/255;c2 = ([120 150 230]+0)/383;c3 = ([120 150 230]+128)/383;patch([0 1 1 0],[0 0 1 1],c1);patch([0 1 1 1-e 1-e 0+e],[0 0 1 1-e 0+e 0+e],c2);patch([0 0 1 1-e 0+e 0+e],[0 1 1 1-e 1-e 0+e],c3);plot([0 1 1 0 0],[0 0 1 1 0]);
  Process Output 1 : Subsystem
      mask Display: e = 0.06;c1 = [120 150 230]/255;c2 = ([120 150 230]+0)/383;c3 = ([120 150 230]+128)/383;patch([0 1 1 0],[0 0 1 1],c1);patch([0 1 1 1-e 1-e 0+e],[0 0 1 1-e 0+e 0+e],c2);patch([0 0 1 1-e 0+e 0+e],[0 1 1 1-e 1-e 0+e],c3);plot([0 1 1 0 0],[0 0 1 1 0]);
  Output : Outport  InitialOutput=[0;0]
      mask Display: e = 0.06;c1 = [120 230 180]/255;c2 = ([120 230 180]+0)/(256+128);c3 = ([120 230 180]+128)/(256+128);patch([0 1 1 0],[0 0 1 1],c1);patch([0 1 1 1-e 1-e 0+e],[0 0 1 1-e 0+e 0+e],c2);patch([0 0 1 1-e 0+e 0+e],[0 1 1 1-e 1-e 0+e],c3);plot([0 1 1 0 0],[0 0 1 1 0]);
  wires:
  Input/1 -> Process Input 1/1(x)
  Process Output 1/1(y) -> Output/1
  Process Input 1/1(p) -> Layer 1/1("p{1}")
  Layer 1/1("a{1}") -> [feedback1]
  [feedback1] -> Layer 2/1("a{1} ")
  Layer 2/1("a{2}") -> Process Output 1/1(a)

== system KiemnghiemDatathudc/network2_6neuron ==
  refx : Inport
  refl : Inport  Port=2
  Demux2 : Demux  Outputs=2
  Fitness APS ZVD4 : Subsystem
  Radians to Degrees4 : simulink_extras/Transformations/Radians to Degrees
  Subsystem5 : Subsystem
  ZVD3 : Subsystem
  network2_6neuron : Subsystem
      mask help: Custom Neural Network
      mask Display: e = 0.06;c1 = [120 150 230]/255;c2 = ([120 150 230]+0)/383;c3 = ([120 150 230]+128)/383;patch([0 1 1 0],[0 0 1 1],c1);patch([0 1 1 1-e 1-e 0+e],[0 0 1 1-e 0+e 0+e],c2);patch([0 0 1 1-e 0+e 0+e],[0 1 1 1-e 1-e 0+e],c3);plot([0 1 1 0 0],[0 0 1 1 0]);fprintf('NNET');port_label('input',1,' Input');port_label('output',1,'Output ');
  Degrees out : Outport
  IAE : Outport  Port=2
  MAx : Outport  Port=3
  x : Outport  Port=4
  l : Outport  Port=5
  wires:
  refl/1 -> Subsystem5/2(ref_ZV1)
  Subsystem5/1(the) -> Radians to Degrees4/1
  Fitness APS ZVD4/1(IAE) -> IAE/1
  Radians to Degrees4/1 -> Degrees out/1, Fitness APS ZVD4/1(e)
  Subsystem5/3(l) -> l/1, network2_6neuron/1(Input)
  Demux2/1 -> ZVD3/2(K)
  ZVD3/1(ref_AZ) -> Subsystem5/1(ref_ZV)  "ref_ZV"
  Demux2/2 -> ZVD3/3(T)
  network2_6neuron/1(Output) -> Demux2/1
  refx/1 -> ZVD3/1(ref)
  Subsystem5/2(x) -> x/1
  Fitness APS ZVD4/2(MAx) -> MAx/1

== system KiemnghiemDatathudc/ANN1/Layer 1 ==
  "p{1}" : Inport  PortDimensions=1
      mask Display: e = 0.06;c1 = [120 230 180]/255;c2 = ([120 230 180]+0)/(256+128);c3 = ([120 230 180]+128)/(256+128);patch([0 1 1 0],[0 0 1 1],c1);patch([0 1 1 1-e 1-e 0+e],[0 0 1 1-e 0+e 0+e],c2);patch([0 0 1 1-e 0+e 0+e],[0 1 1 1-e 1-e 0+e],c3);plot([0 1 1 0 0],[0 0 1 1 0]);
  Delays 1 : Subsystem
      mask Display: e = 0.06;c1 = [120 150 230]/255;c2 = ([120 150 230]+0)/383;c3 = ([120 150 230]+128)/383;patch([0 1 1 0],[0 0 1 1],c1);patch([0 1 1 1-e 1-e 0+e],[0 0 1 1-e 0+e 0+e],c2);patch([0 0 1 1-e 0+e 0+e],[0 1 1 1-e 1-e 0+e],c3);plot([0 1 1 0 0],[0 0 1 1 0]);disp('0');
  "IW{1,1}" : Subsystem
      mask Display: e = 0.06;c1 = [120 150 230]/255;c2 = ([120 150 230]+0)/383;c3 = ([120 150 230]+128)/383;patch([0 1 1 0],[0 0 1 1],c1);patch([0 1 1 1-e 1-e 0+e],[0 0 1 1-e 0+e 0+e],c2);patch([0 0 1 1-e 0+e 0+e],[0 1 1 1-e 1-e 0+e],c3);plot([0 1 1 0 0],[0 0 1 1 0]);disp('W');
  "b{1}" : Constant  Value=[-4.89507064947972647672713719657622277736663818359375;0.81103431841318573969346061858232133090496063232421875;3.73974158150750835005737826577387750148773193359375]
      mask Display: e = 0.06;c1 = [120 150 230]/255;c2 = ([120 150 230]+0)/383;c3 = ([120 150 230]+128)/383;patch([0 1 1 0],[0 0 1 1],c1);patch([0 1 1 1-e 1-e 0+e],[0 0 1 1-e 0+e 0+e],c2);patch([0 0 1 1-e 0+e 0+e],[0 1 1 1-e 1-e 0+e],c3);plot([0 1 1 0 0],[0 0 1 1 0]);disp('b');
  netsum : Sum  Inputs=2  InputSameDT=on  SaturateOnIntegerOverflow=on  OutDataTypeStr=Inherit: Same as first input
      mask Display: e = 0.06;c1 = [120 150 230]/255;c2 = ([120 150 230]+0)/383;c3 = ([120 150 230]+128)/383;patch([0 1 1 0],[0 0 1 1],c1);patch([0 1 1 1-e 1-e 0+e],[0 0 1 1-e 0+e 0+e],c2);patch([0 0 1 1-e 0+e 0+e],[0 1 1 1-e 1-e 0+e],c3);plot([0 1 1 0 0],[0 0 1 1 0]);disp('+');
  tansig : neural/Transfer Functions/tansig
  "a{1}" : Outport  InitialOutput=[0;0;0]
      mask Display: e = 0.06;c1 = [120 230 180]/255;c2 = ([120 230 180]+0)/(256+128);c3 = ([120 230 180]+128)/(256+128);patch([0 1 1 0],[0 0 1 1],c1);patch([0 1 1 1-e 1-e 0+e],[0 0 1 1-e 0+e 0+e],c2);patch([0 0 1 1-e 0+e 0+e],[0 1 1 1-e 1-e 0+e],c3);plot([0 1 1 0 0],[0 0 1 1 0]);
  wires:
  "p{1}"/1 -> Delays 1/1("p{1}")
  Delays 1/1("pd{1,1}") -> "IW{1,1}"/1("pd{1,1}")
  "IW{1,1}"/1("iz{1,1}") -> netsum/1
  "b{1}"/1 -> netsum/2
  netsum/1 -> tansig/1
  tansig/1 -> "a{1}"/1

== system KiemnghiemDatathudc/ANN1/Layer 2 ==
  "a{1} " : Inport  PortDimensions=3
      mask Display: e = 0.06;c1 = [120 230 180]/255;c2 = ([120 230 180]+0)/(256+128);c3 = ([120 230 180]+128)/(256+128);patch([0 1 1 0],[0 0 1 1],c1);patch([0 1 1 1-e 1-e 0+e],[0 0 1 1-e 0+e 0+e],c2);patch([0 0 1 1-e 0+e 0+e],[0 1 1 1-e 1-e 0+e],c3);plot([0 1 1 0 0],[0 0 1 1 0]);
  Delays 1 : Subsystem
      mask Display: e = 0.06;c1 = [120 150 230]/255;c2 = ([120 150 230]+0)/383;c3 = ([120 150 230]+128)/383;patch([0 1 1 0],[0 0 1 1],c1);patch([0 1 1 1-e 1-e 0+e],[0 0 1 1-e 0+e 0+e],c2);patch([0 0 1 1-e 0+e 0+e],[0 1 1 1-e 1-e 0+e],c3);plot([0 1 1 0 0],[0 0 1 1 0]);disp('0');
  "LW{2,1}" : Subsystem
      mask Display: e = 0.06;c1 = [120 150 230]/255;c2 = ([120 150 230]+0)/383;c3 = ([120 150 230]+128)/383;patch([0 1 1 0],[0 0 1 1],c1);patch([0 1 1 1-e 1-e 0+e],[0 0 1 1-e 0+e 0+e],c2);patch([0 0 1 1-e 0+e 0+e],[0 1 1 1-e 1-e 0+e],c3);plot([0 1 1 0 0],[0 0 1 1 0]);disp('W');
  "b{2}" : Constant  Value=[0.0935899089782919746394185267490684054791927337646484375;0.59832509130384126105894893044023774564266204833984375]
      mask Display: e = 0.06;c1 = [120 150 230]/255;c2 = ([120 150 230]+0)/383;c3 = ([120 150 230]+128)/383;patch([0 1 1 0],[0 0 1 1],c1);patch([0 1 1 1-e 1-e 0+e],[0 0 1 1-e 0+e 0+e],c2);patch([0 0 1 1-e 0+e 0+e],[0 1 1 1-e 1-e 0+e],c3);plot([0 1 1 0 0],[0 0 1 1 0]);disp('b');
  netsum : Sum  Inputs=2  InputSameDT=on  SaturateOnIntegerOverflow=on  OutDataTypeStr=Inherit: Same as first input
      mask Display: e = 0.06;c1 = [120 150 230]/255;c2 = ([120 150 230]+0)/383;c3 = ([120 150 230]+128)/383;patch([0 1 1 0],[0 0 1 1],c1);patch([0 1 1 1-e 1-e 0+e],[0 0 1 1-e 0+e 0+e],c2);patch([0 0 1 1-e 0+e 0+e],[0 1 1 1-e 1-e 0+e],c3);plot([0 1 1 0 0],[0 0 1 1 0]);disp('+');
  purelin : neural/Transfer Functions/purelin
  "a{2}" : Outport  InitialOutput=[0;0]
      mask Display: e = 0.06;c1 = [120 230 180]/255;c2 = ([120 230 180]+0)/(256+128);c3 = ([120 230 180]+128)/(256+128);patch([0 1 1 0],[0 0 1 1],c1);patch([0 1 1 1-e 1-e 0+e],[0 0 1 1-e 0+e 0+e],c2);patch([0 0 1 1-e 0+e 0+e],[0 1 1 1-e 1-e 0+e],c3);plot([0 1 1 0 0],[0 0 1 1 0]);
  wires:
  "a{1} "/1 -> Delays 1/1("p{2}")
  Delays 1/1("pd{2,1}") -> "LW{2,1}"/1("ad{2,1}")
  "LW{2,1}"/1("lz{2,1}") -> netsum/1
  "b{2}"/1 -> netsum/2
  netsum/1 -> purelin/1
  purelin/1 -> "a{2}"/1

== system KiemnghiemDatathudc/ANN1/Process Input 1 ==
  x : Inport  PortDimensions=1
      mask Display: e = 0.06;c1 = [120 230 180]/255;c2 = ([120 230 180]+0)/(256+128);c3 = ([120 230 180]+128)/(256+128);patch([0 1 1 0],[0 0 1 1],c1);patch([0 1 1 1-e 1-e 0+e],[0 0 1 1-e 0+e 0+e],c2);patch([0 0 1 1-e 0+e 0+e],[0 1 1 1-e 1-e 0+e],c3);plot([0 1 1 0 0],[0 0 1 1 0]);
  mapminmax : neural/Processing Functions/mapminmax  xmin=0.400000000000000022204460492503  xmax=0.599999999999999977795539507497  ymin=-1  ymax=1
  p : Outport  PortDimensions=1
      mask Display: e = 0.06;c1 = [120 230 180]/255;c2 = ([120 230 180]+0)/(256+128);c3 = ([120 230 180]+128)/(256+128);patch([0 1 1 0],[0 0 1 1],c1);patch([0 1 1 1-e 1-e 0+e],[0 0 1 1-e 0+e 0+e],c2);patch([0 0 1 1-e 0+e 0+e],[0 1 1 1-e 1-e 0+e],c3);plot([0 1 1 0 0],[0 0 1 1 0]);
  wires:
  x/1 -> mapminmax/1
  mapminmax/1 -> p/1

== system KiemnghiemDatathudc/ANN1/Process Output 1 ==
  a : Inport  PortDimensions=2
      mask Display: e = 0.06;c1 = [120 230 180]/255;c2 = ([120 230 180]+0)/(256+128);c3 = ([120 230 180]+128)/(256+128);patch([0 1 1 0],[0 0 1 1],c1);patch([0 1 1 1-e 1-e 0+e],[0 0 1 1-e 0+e 0+e],c2);patch([0 0 1 1-e 0+e 0+e],[0 1 1 1-e 1-e 0+e],c3);plot([0 1 1 0 0],[0 0 1 1 0]);
  mapminmax_reverse : neural/Processing Functions/mapminmax_reverse  xmin=[0.891093182220120016978626154014;0.791266899561214986924539971369]  xmax=[0.947329586635518028359115305648;0.803724881678661962070009394665]  ymin=-1  ymax=1
  y : Outport  PortDimensions=2
      mask Display: e = 0.06;c1 = [120 230 180]/255;c2 = ([120 230 180]+0)/(256+128);c3 = ([120 230 180]+128)/(256+128);patch([0 1 1 0],[0 0 1 1],c1);patch([0 1 1 1-e 1-e 0+e],[0 0 1 1-e 0+e 0+e],c2);patch([0 0 1 1-e 0+e 0+e],[0 1 1 1-e 1-e 0+e],c3);plot([0 1 1 0 0],[0 0 1 1 0]);
  wires:
  a/1 -> mapminmax_reverse/1
  mapminmax_reverse/1 -> y/1

== system KiemnghiemDatathudc/AOL/AOL ==
  ref : Inport
  Gain : Gain  Gain=0.25
  Gain1 : Gain  Gain=0.5
  Gain2 : Gain  Gain=0.25
  Sum : Sum  Inputs=+++
  Transport Delay : TransportDelay  DelayTime=pi/waol
  Transport Delay1 : TransportDelay  DelayTime=2*pi/waol
  ref_AZ : Outport
  wires:
  Gain1/1 -> Transport Delay/1
  Gain/1 -> Sum/1
  Transport Delay/1 -> Sum/2
  Sum/1 -> ref_AZ/1
  ref/1 -> Gain/1, Gain2/1, Gain1/1
  Gain2/1 -> Transport Delay1/1
  Transport Delay1/1 -> Sum/3

== system KiemnghiemDatathudc/AOL/Fitness APS ZVD4 ==
  e : Inport
  Abs : Abs
  Abs1 : Abs
  Integrator : Integrator
  MinMax Running Resettable : simulink/Math Operations/MinMax Running Resettable  Function=max  vinit=0.0
  Step : Step  Time=0.000001  Before=1  After=0  SampleTime=0
  IAE : Outport
  MAx : Outport  Port=2
  wires:
  Abs/1 -> Integrator/1
  Abs1/1 -> MinMax Running Resettable/1
  Step/1 -> MinMax Running Resettable/2
  e/1 -> Abs/1, Abs1/1
  Integrator/1 -> IAE/1
  MinMax Running Resettable/1 -> MAx/1

== system KiemnghiemDatathudc/AOL/Subsystem5 ==
  ref_ZV : Inport
  ref_ZV1 : Inport  Port=2
  "ADRC " : Subsystem
  ADRC 1 : Subsystem
  Constant : Constant  Value=mc
  Gain : Gain  Gain=1/3
  Scope : Scope
  Subsystem : Subsystem
  the : Outport
  x : Outport  Port=2
  l : Outport  Port=3
  wires:
  Subsystem/1(x) -> x/1, "ADRC "/2(x)  "Position"
  ADRC 1/1(u) -> Subsystem/2(ul)  "ADRC"
  Subsystem/3(the) -> Gain/1
  Subsystem/2(l) -> l/1, Scope/1, ADRC 1/2(x)  "Length"
  "ADRC "/1(u) -> Subsystem/1(ut)  "ADRC"
  ref_ZV1/1 -> ADRC 1/1(ref)
  ref_ZV/1 -> "ADRC "/1(ref)
  Gain/1 -> the/1
  Constant/1 -> Subsystem/3(mc)

== system KiemnghiemDatathudc/Subsystem/AOF ==
  ref : Inport
  Gain : Gain  Gain=0.25
  Gain1 : Gain  Gain=0.5
  Gain2 : Gain  Gain=0.25
  Sum : Sum  Inputs=+++
  Transport Delay : TransportDelay  DelayTime=pi/waof
  Transport Delay1 : TransportDelay  DelayTime=2*pi/waof
  ref_AZ : Outport
  wires:
  Gain1/1 -> Transport Delay/1
  Gain/1 -> Sum/1
  Transport Delay/1 -> Sum/2
  Sum/1 -> ref_AZ/1
  ref/1 -> Gain/1, Gain2/1, Gain1/1
  Gain2/1 -> Transport Delay1/1
  Transport Delay1/1 -> Sum/3

== system KiemnghiemDatathudc/Subsystem/AOF2 ==
  ref : Inport
  Gain : Gain  Gain=0.25
  Gain1 : Gain  Gain=0.5
  Gain2 : Gain  Gain=0.25
  Sum : Sum  Inputs=+++
  Transport Delay : TransportDelay  DelayTime=pi/waof
  Transport Delay1 : TransportDelay  DelayTime=2*pi/waof
  ref_AZ : Outport
  wires:
  Gain1/1 -> Transport Delay/1
  Gain/1 -> Sum/1
  Transport Delay/1 -> Sum/2
  Sum/1 -> ref_AZ/1
  ref/1 -> Gain/1, Gain2/1, Gain1/1
  Gain2/1 -> Transport Delay1/1
  Transport Delay1/1 -> Sum/3

== system KiemnghiemDatathudc/Subsystem/Fitness APS ZVD1 ==
  e : Inport
  Abs : Abs
  Abs1 : Abs
  Integrator : Integrator
  MinMax Running Resettable : simulink/Math Operations/MinMax Running Resettable  Function=max  vinit=0.0
  Step : Step  Time=0.000001  Before=1  After=0  SampleTime=0
  IAE : Outport
  MAx : Outport  Port=2
  wires:
  Abs/1 -> Integrator/1
  Abs1/1 -> MinMax Running Resettable/1
  Step/1 -> MinMax Running Resettable/2
  e/1 -> Abs/1, Abs1/1
  Integrator/1 -> IAE/1
  MinMax Running Resettable/1 -> MAx/1

== system KiemnghiemDatathudc/Subsystem/Subsystem5 ==
  ref_ZV : Inport
  ref_ZV1 : Inport  Port=2
  "ADRC " : Subsystem
  ADRC 1 : Subsystem
  Constant : Constant  Value=mc
  Gain : Gain  Gain=1/3
  Subsystem : Subsystem
  the : Outport
  x : Outport  Port=2
  l : Outport  Port=3
  wires:
  Subsystem/1(x) -> x/1, "ADRC "/2(x)  "Position"
  ADRC 1/1(u) -> Subsystem/2(ul)  "ADRC"
  Subsystem/3(the) -> Gain/1
  Subsystem/2(l) -> ADRC 1/2(x), l/1  "Length"
  "ADRC "/1(u) -> Subsystem/1(ut)  "ADRC"
  ref_ZV1/1 -> ADRC 1/1(ref)
  ref_ZV/1 -> "ADRC "/1(ref)
  Gain/1 -> the/1
  Constant/1 -> Subsystem/3(mc)

== system KiemnghiemDatathudc/Subsystem1/ADRC  ==
  ref : Inport
  x : Inport  Port=2
  Gain : Gain  Gain=Kp
  Gain1 : Gain  Gain=Kd
  Gain2 : Gain  Gain=1/b0
  Observer : Subsystem
  Sum : Sum  Inputs=|+-
  Sum3 : Sum  Inputs=|+-
  Sum4 : Sum  Inputs=|+-
  u : Outport
  wires:
  Sum4/1 -> Gain2/1
  Sum/1 -> Gain/1
  Gain2/1 -> u/1, Observer/1(u)
  x/1 -> Observer/2(x)
  Sum3/1 -> Sum4/1
  Observer/2(x2) -> Gain1/1
  Gain1/1 -> Sum3/2
  Gain/1 -> Sum3/1
  ref/1 -> Sum/1
  Observer/1(x3) -> Sum4/2
  Observer/3(x1) -> Sum/2

== system KiemnghiemDatathudc/Subsystem1/ADRC 1 ==
  ref : Inport
  x : Inport  Port=2
  Gain : Gain  Gain=Kp1
  Gain1 : Gain  Gain=Kd1
  Gain2 : Gain  Gain=1/b1
  Observer : Subsystem
  Sum : Sum  Inputs=|+-
  Sum3 : Sum  Inputs=|+-
  Sum4 : Sum  Inputs=|+-
  u : Outport
  wires:
  Sum4/1 -> Gain2/1
  Sum/1 -> Gain/1
  Gain2/1 -> u/1, Observer/1(u)
  x/1 -> Observer/2(x)
  Sum3/1 -> Sum4/1
  Observer/2(x2) -> Gain1/1
  Gain1/1 -> Sum3/2
  Gain/1 -> Sum3/1
  ref/1 -> Sum/1
  Observer/1(x3) -> Sum4/2
  Observer/3(x1) -> Sum/2

== system KiemnghiemDatathudc/Subsystem1/Subsystem ==
  ut : Inport
  ul : Inport  Port=2
  mc : Inport  Port=3
  Add : Sum
  Constant : Constant  Value=-mc*g
  Crane : MATLAB Function  TreatAsAtomicUnit=on
  Integrator{,1,3..5} (5 alike) : Integrator
  Integrator2 : Integrator  InitialCondition=l_ini
  x : Outport
  l : Outport  Port=2
  the : Outport  Port=3
  wires:
  Integrator5/1 -> [x6]
  Integrator2/1 -> l/1, [x3]
  [x4] -> Crane/4(x4)
  Crane/5(dx5) -> Integrator4/1
  Crane/6(dx6) -> Integrator5/1
  Crane/1(dx1) -> Integrator/1
  Crane/3(dx3) -> Integrator2/1
  Integrator1/1 -> [x2]
  [x2] -> Crane/2(x2)
  Integrator4/1 -> the/1, [x5]
  [x3] -> Crane/3(x3)
  [x6] -> Crane/6(x6)
  [x5] -> Crane/5(x5)
  Crane/4(dx4) -> Integrator3/1
  Integrator/1 -> x/1, [x1]
  Integrator3/1 -> [x4]
  [x1] -> Crane/1(x1)
  Crane/2(dx2) -> Integrator1/1
  ut/1 -> Crane/7(ut)
  ul/1 -> Add/2
  Constant/1 -> Add/1
  Add/1 -> Crane/8(ul)
  mc/1 -> Crane/9(mc)

== system KiemnghiemDatathudc/Subsystem2/AOF ==
  ref : Inport
  Gain : Gain  Gain=0.25
  Gain1 : Gain  Gain=0.5
  Gain2 : Gain  Gain=0.25
  Sum : Sum  Inputs=+++
  Transport Delay : TransportDelay  DelayTime=pi/waof
  Transport Delay1 : TransportDelay  DelayTime=2*pi/waof
  ref_AZ : Outport
  wires:
  Gain1/1 -> Transport Delay/1
  Gain/1 -> Sum/1
  Transport Delay/1 -> Sum/2
  Sum/1 -> ref_AZ/1
  ref/1 -> Gain/1, Gain2/1, Gain1/1
  Gain2/1 -> Transport Delay1/1
  Transport Delay1/1 -> Sum/3

== system KiemnghiemDatathudc/Subsystem2/Fitness APS ZVD1 ==
  e : Inport
  Abs : Abs
  Abs1 : Abs
  Integrator : Integrator
  MinMax Running Resettable : simulink/Math Operations/MinMax Running Resettable  Function=max  vinit=0.0
  Step : Step  Time=0.000001  Before=1  After=0  SampleTime=0
  IAE : Outport
  MAx : Outport  Port=2
  wires:
  Abs/1 -> Integrator/1
  Abs1/1 -> MinMax Running Resettable/1
  Step/1 -> MinMax Running Resettable/2
  e/1 -> Abs/1, Abs1/1
  Integrator/1 -> IAE/1
  MinMax Running Resettable/1 -> MAx/1

== system KiemnghiemDatathudc/Subsystem2/Subsystem5 ==
  ref_ZV : Inport
  ref_ZV1 : Inport  Port=2
  "ADRC " : Subsystem
  ADRC 1 : Subsystem
  Constant : Constant  Value=mc
  Gain : Gain  Gain=1/3
  Subsystem : Subsystem
  the : Outport
  x : Outport  Port=2
  l : Outport  Port=3
  wires:
  Subsystem/1(x) -> x/1, "ADRC "/2(x)  "Position"
  ADRC 1/1(u) -> Subsystem/2(ul)  "ADRC"
  Subsystem/3(the) -> Gain/1
  Subsystem/2(l) -> ADRC 1/2(x), l/1  "Length"
  "ADRC "/1(u) -> Subsystem/1(ut)  "ADRC"
  ref_ZV1/1 -> ADRC 1/1(ref)
  ref_ZV/1 -> "ADRC "/1(ref)
  Gain/1 -> the/1
  Constant/1 -> Subsystem/3(mc)

== system KiemnghiemDatathudc/data_l_conzv_3neuron1/Custom Neural Network1 ==
  Input : Inport  PortDimensions=1
      mask Display: e = 0.06;c1 = [120 230 180]/255;c2 = ([120 230 180]+0)/(256+128);c3 = ([120 230 180]+128)/(256+128);patch([0 1 1 0],[0 0 1 1],c1);patch([0 1 1 1-e 1-e 0+e],[0 0 1 1-e 0+e 0+e],c2);patch([0 0 1 1-e 0+e 0+e],[0 1 1 1-e 1-e 0+e],c3);plot([0 1 1 0 0],[0 0 1 1 0]);
  Layer 1 : Subsystem
      mask Display: e = 0.06;c1 = [120 150 230]/255;c2 = ([120 150 230]+0)/383;c3 = ([120 150 230]+128)/383;patch([0 1 1 0],[0 0 1 1],c1);patch([0 1 1 1-e 1-e 0+e],[0 0 1 1-e 0+e 0+e],c2);patch([0 0 1 1-e 0+e 0+e],[0 1 1 1-e 1-e 0+e],c3);plot([0 1 1 0 0],[0 0 1 1 0]);
  Layer 2 : Subsystem
      mask Display: e = 0.06;c1 = [120 150 230]/255;c2 = ([120 150 230]+0)/383;c3 = ([120 150 230]+128)/383;patch([0 1 1 0],[0 0 1 1],c1);patch([0 1 1 1-e 1-e 0+e],[0 0 1 1-e 0+e 0+e],c2);patch([0 0 1 1-e 0+e 0+e],[0 1 1 1-e 1-e 0+e],c3);plot([0 1 1 0 0],[0 0 1 1 0]);
  Process Input 1 : Subsystem
      mask Display: e = 0.06;c1 = [120 150 230]/255;c2 = ([120 150 230]+0)/383;c3 = ([120 150 230]+128)/383;patch([0 1 1 0],[0 0 1 1],c1);patch([0 1 1 1-e 1-e 0+e],[0 0 1 1-e 0+e 0+e],c2);patch([0 0 1 1-e 0+e 0+e],[0 1 1 1-e 1-e 0+e],c3);plot([0 1 1 0 0],[0 0 1 1 0]);
  Process Output 1 : Subsystem
      mask Display: e = 0.06;c1 = [120 150 230]/255;c2 = ([120 150 230]+0)/383;c3 = ([120 150 230]+128)/383;patch([0 1 1 0],[0 0 1 1],c1);patch([0 1 1 1-e 1-e 0+e],[0 0 1 1-e 0+e 0+e],c2);patch([0 0 1 1-e 0+e 0+e],[0 1 1 1-e 1-e 0+e],c3);plot([0 1 1 0 0],[0 0 1 1 0]);
  Output : Outport  InitialOutput=0
      mask Display: e = 0.06;c1 = [120 230 180]/255;c2 = ([120 230 180]+0)/(256+128);c3 = ([120 230 180]+128)/(256+128);patch([0 1 1 0],[0 0 1 1],c1);patch([0 1 1 1-e 1-e 0+e],[0 0 1 1-e 0+e 0+e],c2);patch([0 0 1 1-e 0+e 0+e],[0 1 1 1-e 1-e 0+e],c3);plot([0 1 1 0 0],[0 0 1 1 0]);
  wires:
  Input/1 -> Process Input 1/1(x)
  Process Output 1/1(y) -> Output/1
  Process Input 1/1(p) -> Layer 1/1("p{1}")
  Layer 1/1("a{1}") -> [feedback1]
  [feedback1] -> Layer 2/1("a{1} ")
  Layer 2/1("a{2}") -> Process Output 1/1(a)

== system KiemnghiemDatathudc/data_l_conzv_3neuron1/Fitness APS ZVD4 ==
  e : Inport
  Abs : Abs
  Abs1 : Abs
  Integrator : Integrator
  MinMax Running Resettable : simulink/Math Operations/MinMax Running Resettable  Function=max  vinit=0.0
  Step : Step  Time=0.000001  Before=1  After=0  SampleTime=0
  IAE : Outport
  MAx : Outport  Port=2
  wires:
  Abs/1 -> Integrator/1
  Abs1/1 -> MinMax Running Resettable/1
  Step/1 -> MinMax Running Resettable/2
  e/1 -> Abs/1, Abs1/1
  Integrator/1 -> IAE/1
  MinMax Running Resettable/1 -> MAx/1

== system KiemnghiemDatathudc/data_l_conzv_3neuron1/Subsystem5 ==
  ref_ZV : Inport
  ref_ZV1 : Inport  Port=2
  "ADRC " : Subsystem
  ADRC 1 : Subsystem
  Constant : Constant  Value=mc
  Gain : Gain  Gain=1/3
  Subsystem : Subsystem
  the : Outport
  x : Outport  Port=2
  l : Outport  Port=3
  wires:
  Subsystem/1(x) -> x/1, "ADRC "/2(x)  "Position"
  ADRC 1/1(u) -> Subsystem/2(ul)  "ADRC"
  Subsystem/3(the) -> Gain/1
  Subsystem/2(l) -> ADRC 1/2(x), l/1  "Length"
  "ADRC "/1(u) -> Subsystem/1(ut)  "ADRC"
  ref_ZV1/1 -> ADRC 1/1(ref)
  ref_ZV/1 -> "ADRC "/1(ref)
  Gain/1 -> the/1
  Constant/1 -> Subsystem/3(mc)

== system KiemnghiemDatathudc/data_l_conzv_3neuron1/ZV3 ==
  ref : Inport
  Input : Inport  Port=2
  Gain1 : Gain  Gain=0.5
  Gain2 : Gain  Gain=0.5
  Sum : Sum
  Variable Transport Delay : VariableTransportDelay  VariableDelayType=Variable transport delay  MaximumDelay=10
  ref_AZ : Outport
  wires:
  Gain2/1 -> Variable Transport Delay/1
  Gain1/1 -> Sum/1
  Variable Transport Delay/1 -> Sum/2
  Sum/1 -> ref_AZ/1
  ref/1 -> Gain1/1, Gain2/1
  Input/1 -> Variable Transport Delay/2
